simulink model "CopterSim3DEnvironment"  (R2017b)
settings: Solver=ode4  StartTime=0.0  StopTime=2000  FixedStep=0.001  RelTol=1e-3
PreLoadFcn:
  | filepath  = fileparts(get_param(bdroot, 'FileName'))
  | cd(filepath);
InitFcn:
  | if exist('Init_control.m','file')
  |      Init_control;
  | end
values from neighbouring files (symbols this model uses):
  Kd_RP_AgngleRate = 0.005    [Init_control.m]
  Kd_YAW_AngleRate = 0.05    [Init_control.m]
  Ki_RP_AgngleRate = 0.01    [Init_control.m]
  Ki_YAW_AngleRate = 0.8    [Init_control.m]
  Kp_RP_AgngleRate = 0.55    [Init_control.m]
  Kp_RP_ANGLE = 6.5    [Init_control.m]
  Kp_YAW_AngleRate = 3.2    [Init_control.m]
  MAX_CONTROL_ANGLE_RATE_Y = 90    [Init_control.m]
  MAX_CONTROL_ANGLE_RP = 45    [Init_control.m]
undefined symbols (not defined in the file or in its folder): earthRadius, KiPitchAttitude, KiRollAttitude, ModelInit_RPM, ModelParam_envAltitude, ModelParam_GlobalNoiseGainSwitch, ModelParam_GPSLatLong, ModelParam_motorCr, ModelParam_motorJm, ModelParam_motorMinThr, ModelParam_motorT, ModelParam_motorWb, ModelParam_rotorCm, ModelParam_rotorCt, ModelParam_uavCCm, ModelParam_uavCd, ModelParam_uavDearo, ModelParam_uavJ, ModelParam_uavMass, ModelParam_uavR, ModelParam_uavType, Receive, Send
libraries: simulink x6, aerolibfltsims x4, etargetslib x2, shared6dof x1, aerolibanimutils x1, dspnetwork x1
(part 1 of 2)
settings Model: SimulationMode=accelerator  Creator=dream  LastModifiedBy=dream
settings DebuggingCC: BusObjectLabelMismatch=error
settings CodeAppCC: StateflowObjectComments=on

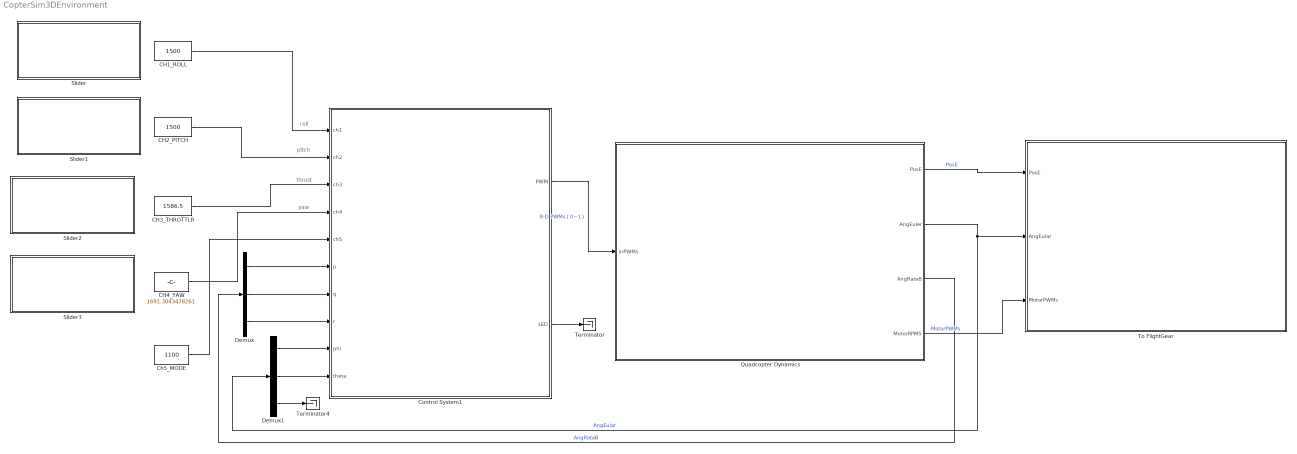
== system CopterSim3DEnvironment ==
  note: roll
  note: pitch
  note: thrust
  note: yaw
  "     CH3_THROTTLR " : Constant  Value=1586.5  OutDataTypeStr=uint16
  "     CH4_YAW     " : Constant  Value=1691.3043478261  OutDataTypeStr=uint16
  " CH2_PITCH " : Constant  Value=1500  OutDataTypeStr=uint16
  "CH1_ROLL   " : Constant  Value=1500  OutDataTypeStr=uint16
  "Ch5_MODE " : Constant  Value=1100  OutDataTypeStr=uint16
  Control System1 : Subsystem
      mask Display: image('icon\pixhawk.png');
  Demux : Demux  Outputs=3
  Demux1 : Demux  Outputs=3
  Quadcopter Dynamics : Subsystem
      mask Display: image('icon/F450.png');
  Slider : Subsystem  DialogController=hmiCreateDDGDialog  IsWebBlock=on  mask(MWDashboardBlock){webBlockId=da57f061-4e57-426f-be23-e227219c210b, webBlockType=slider, ShowInLibBrowser=on, ShowInitialText=on, HMISrcModelName=CopterSim3DEnvironment}
      mask prompts: webBlockId "WebBlock Id"; webBlockType "WebBlock Type"; HMISrcModelName "Source Model"
      mask help: SimulinkHMI:dialogs:SliderDialogDesc
      mask Help: helpview([docroot '/mapfiles/simulink.map'], 'hmi_slider')
      mask Display:
      | if strcmp(get_param(bdroot(gcb),'BlockDiagramType'), 'library')
      |     image([(matlabroot) '/toolbox/simulink/hmi/icons/Slider.png']);
      | end
  Slider1 : Subsystem  DialogController=hmiCreateDDGDialog  IsWebBlock=on  mask(MWDashboardBlock){webBlockId=f8138af1-f0d8-4bb2-b2ca-4a41ecd2e2bf, webBlockType=slider, ShowInLibBrowser=on, ShowInitialText=on, HMISrcModelName=CopterSim3DEnvironment}
      mask prompts: webBlockId "WebBlock Id"; webBlockType "WebBlock Type"; HMISrcModelName "Source Model"
      mask help: SimulinkHMI:dialogs:SliderDialogDesc
      mask Help: helpview([docroot '/mapfiles/simulink.map'], 'hmi_slider')
      mask Display:
      | if strcmp(get_param(bdroot(gcb),'BlockDiagramType'), 'library')
      |     image([(matlabroot) '/toolbox/simulink/hmi/icons/Slider.png']);
      | end
  Slider2 : Subsystem  DialogController=hmiCreateDDGDialog  IsWebBlock=on  mask(MWDashboardBlock){webBlockId=6ace0251-812b-4be1-a029-ff54be59cd06, webBlockType=slider, ShowInLibBrowser=on, ShowInitialText=on, HMISrcModelName=CopterSim3DEnvironment}
      mask prompts: webBlockId "WebBlock Id"; webBlockType "WebBlock Type"; HMISrcModelName "Source Model"
      mask help: SimulinkHMI:dialogs:SliderDialogDesc
      mask Help: helpview([docroot '/mapfiles/simulink.map'], 'hmi_slider')
      mask Display:
      | if strcmp(get_param(bdroot(gcb),'BlockDiagramType'), 'library')
      |     image([(matlabroot) '/toolbox/simulink/hmi/icons/Slider.png']);
      | end
  Slider3 : Subsystem  DialogController=hmiCreateDDGDialog  IsWebBlock=on  mask(MWDashboardBlock){webBlockId=7791c665-d291-46cf-a452-489177f2fb62, webBlockType=slider, ShowInLibBrowser=on, ShowInitialText=on, HMISrcModelName=CopterSim3DEnvironment}
      mask prompts: webBlockId "WebBlock Id"; webBlockType "WebBlock Type"; HMISrcModelName "Source Model"
      mask help: SimulinkHMI:dialogs:SliderDialogDesc
      mask Help: helpview([docroot '/mapfiles/simulink.map'], 'hmi_slider')
      mask Display:
      | if strcmp(get_param(bdroot(gcb),'BlockDiagramType'), 'library')
      |     image([(matlabroot) '/toolbox/simulink/hmi/icons/Slider.png']);
      | end
  Terminator : Terminator
  Terminator4 : Terminator
  To FlightGear : Subsystem
      mask Display: image('icon/FlightGear.png');
  wires:
  Quadcopter Dynamics/1(PosE) -> To FlightGear/1(PosE)  "PosE"
  Control System1/2(LED) -> Terminator/1
  Quadcopter Dynamics/2(AngEuler) -> To FlightGear/2(AngEular), Demux1/1  "AngEular"
  "CH1_ROLL   "/1 -> Control System1/1(ch1)
  "     CH4_YAW     "/1 -> Control System1/4(ch4)
  "     CH3_THROTTLR "/1 -> Control System1/3(ch3)
  Quadcopter Dynamics/3(AngRateB) -> Demux/1  "AngRateB"
  "Ch5_MODE "/1 -> Control System1/5(ch5)
  Demux/1 -> Control System1/6(p)
  Demux/2 -> Control System1/7(q)
  Demux/3 -> Control System1/8(r)
  Demux1/1 -> Control System1/9(phi)
  Demux1/2 -> Control System1/10(theta)
  Demux1/3 -> Terminator4/1
  " CH2_PITCH "/1 -> Control System1/2(ch2)
  Control System1/1(PWM) -> Quadcopter Dynamics/1(inPWMs)  "8-D PWMs（0~1）"
  Quadcopter Dynamics/4(MotorRPMS) -> To FlightGear/3(MotorPWMs)  "MotorPWMs"

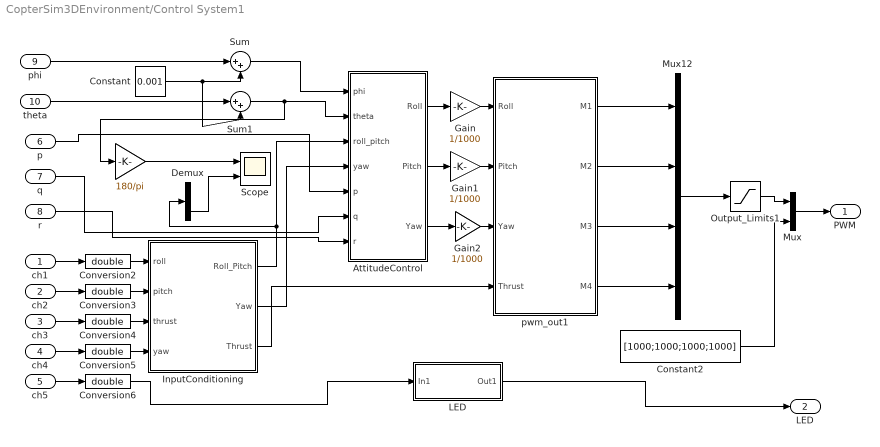
== system CopterSim3DEnvironment/Control System1 ==
  ch1 : Inport  OutDataTypeStr=uint16  PortDimensions=1
  ch2 : Inport  Port=2  OutDataTypeStr=uint16  PortDimensions=1
  ch3 : Inport  Port=3  OutDataTypeStr=uint16  PortDimensions=1
  ch4 : Inport  Port=4  OutDataTypeStr=uint16  PortDimensions=1
  ch5 : Inport  Port=5  OutDataTypeStr=uint16  PortDimensions=1  Interpolate=off
  p : Inport  Port=6  PortDimensions=1
  q : Inport  Port=7  PortDimensions=1
  r : Inport  Port=8  PortDimensions=1
  phi : Inport  Port=9  PortDimensions=1
  theta : Inport  Port=10  PortDimensions=1
  " " : Gain  Gain=180/pi
  AttitudeControl : Subsystem
  Constant : Constant  Value=0.001
  Constant2 : Constant  Value=[1000;1000;1000;1000]
  Conversion{2..6} (5 alike) : DataTypeConversion  OutDataTypeStr=double
  Demux : Demux  Outputs=2
  Gain : Gain  Gain=1/1000
  Gain1 : Gain  Gain=1/1000
  Gain2 : Gain  Gain=1/1000
  InputConditioning : Subsystem
  "LED " : Subsystem
  Mux : Mux  Inputs=2
  Mux12 : Mux
  Output_Limits1 : Saturate  UpperLimit=2000  LowerLimit=1000
  Scope : Scope  NumInputPorts=2
  Sum : Sum  Inputs=|++
  Sum1 : Sum  Inputs=|++
  pwm_out1 : MATLAB Function  TreatAsAtomicUnit=on  SystemSampleTime=0.004
  PWM : Outport  PortDimensions=8
  LED : Outport  Port=2  PortDimensions=1
  wires:
  InputConditioning/3(Thrust) -> pwm_out1/4(Thrust)
  Mux12/1 -> Output_Limits1/1
  Gain1/1 -> pwm_out1/2(Pitch)
  Gain/1 -> pwm_out1/1(Roll)
  ch3/1 -> Conversion4/1
  pwm_out1/1(M1) -> Mux12/1
  ch5/1 -> Conversion6/1
  pwm_out1/3(M3) -> Mux12/3
  pwm_out1/2(M2) -> Mux12/2
  r/1 -> AttitudeControl/7(r)
  AttitudeControl/1(Roll) -> Gain/1
  Gain2/1 -> pwm_out1/3(Yaw)
  InputConditioning/1(Roll_Pitch) -> Demux/1, AttitudeControl/3(roll_pitch)
  q/1 -> AttitudeControl/6(q)
  theta/1 -> Sum1/1
  InputConditioning/2(Yaw) -> AttitudeControl/4(yaw)
  p/1 -> AttitudeControl/5(p)
  ch4/1 -> Conversion5/1
  pwm_out1/4(M4) -> Mux12/4
  AttitudeControl/3(Yaw) -> Gain2/1
  AttitudeControl/2(Pitch) -> Gain1/1
  ch1/1 -> Conversion2/1
  "LED "/1(Out1) -> LED/1
  ch2/1 -> Conversion3/1
  Conversion6/1 -> "LED "/1(In1)
  Conversion2/1 -> InputConditioning/1(roll)
  Conversion5/1 -> InputConditioning/4(yaw)
  Conversion4/1 -> InputConditioning/3(thrust)
  Conversion3/1 -> InputConditioning/2(pitch)
  " "/1 -> Scope/1
  Demux/2 -> Scope/2
  phi/1 -> Sum/1
  Sum/1 -> AttitudeControl/1(phi)
  Sum1/1 -> " "/1, AttitudeControl/2(theta)
  Constant/1 -> Sum1/2, Sum/2
  Constant2/1 -> Mux/2
  Output_Limits1/1 -> Mux/1
  Mux/1 -> PWM/1

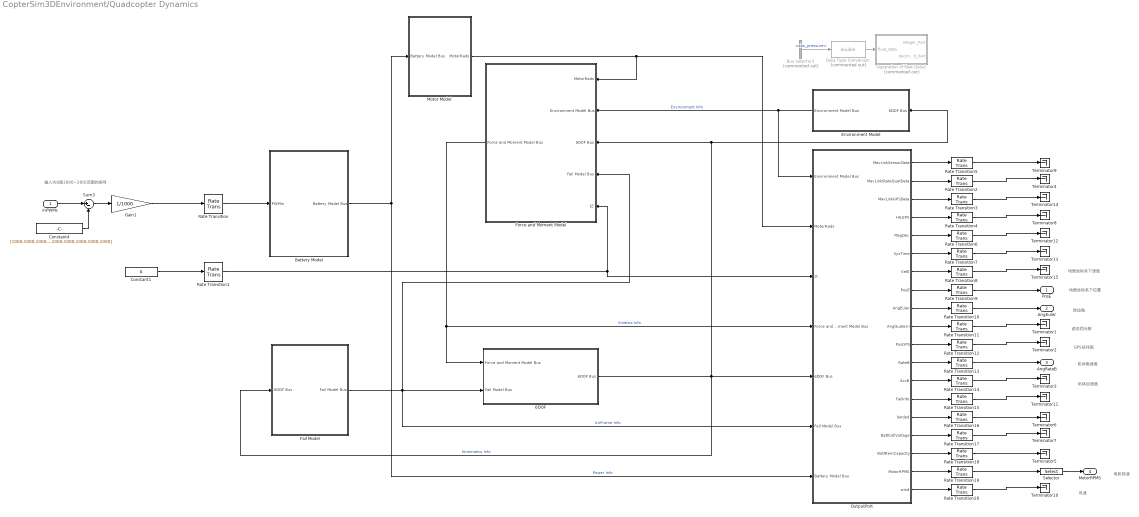
== system CopterSim3DEnvironment/Quadcopter Dynamics ==
  note: 电机转速
  note: 风速
  note: 机体加速度
  note: 机体角速度
  note: GPS经纬高
  note: 姿态四元数
  note: 欧拉角
  note: 地面坐标系下位置
  note: 地面坐标系下速度
  note: 输入为8路1000~2000范围的信号
  inPWMs : Inport  PortDimensions=8
  6DOF : Subsystem
  Battery Model : Subsystem
      mask help: Simulink:masks:GenSFuncDesc_MD
      mask Help: eval('feval(''rtwprivate'',''rtwhelpview'',''rtw_sfcn_block'')');
  Bus Selector3 : BusSelector  Commented=on  OutputSignals=abs_pressure
  Constant1 : Constant  Value=0
  Constant4 : Constant  Value=[1000;1000;1000;1000;1000;1000;1000;1000]
  Data Type Conversion : DataTypeConversion  Commented=on  OutDataTypeStr=double
  Environment Model : Subsystem  mask{sfcnParam1=ModelParam_GPSLatLong, sfcnParam2=ModelParam_GlobalNoiseGainSwitch, sfcnParam3=ModelParam_envAltitude}
      mask prompts: sfcnParam1 "ModelParam_GPSLatLong:"; sfcnParam2 "ModelParam_GlobalNoiseGainSwitch:"; sfcnParam3 "ModelParam_envAltitude:"
      mask help: Simulink:masks:GenSFuncDesc_MD
      mask Help: eval('feval(''rtwprivate'',''rtwhelpview'',''rtw_sfcn_block'')');
  Fail Model : Subsystem  mask{sfcnParam1=ModelParam_uavJ, sfcnParam2=ModelParam_uavMass, sfcnParam3=ModelParam_uavR}
      mask prompts: sfcnParam1 "ModelParam_uavJ:"; sfcnParam2 "ModelParam_uavMass:"; sfcnParam3 "ModelParam_uavR:"
      mask help: Simulink:masks:GenSFuncDesc_MD
      mask Help: eval('feval(''rtwprivate'',''rtwhelpview'',''rtw_sfcn_block'')');
  Force and Moment Model : Subsystem  mask{sfcnParam1=ModelParam_motorJm, sfcnParam2=ModelParam_rotorCm, sfcnParam3=ModelParam_rotorCt, sfcnParam4=ModelParam_uavCCm, sfcnParam5=ModelParam_uavCd, sfcnParam6=ModelParam_uavDearo, sfcnParam7=ModelParam_uavR, sfcnParam8=ModelParam_uavType}
      mask prompts: sfcnParam1 "ModelParam_motorJm:"; sfcnParam2 "ModelParam_rotorCm:"; sfcnParam3 "ModelParam_rotorCt:"; sfcnParam4 "ModelParam_uavCCm:"; sfcnParam5 "ModelParam_uavCd:"; sfcnParam6 "ModelParam_uavDearo:"; sfcnParam7 "ModelParam_uavR:"; sfcnParam8 "ModelParam_uavType:"
      mask help: Simulink:masks:GenSFuncDesc_MD
      mask Help: eval('feval(''rtwprivate'',''rtwhelpview'',''rtw_sfcn_block'')');
  Gain1 : Gain  Gain=1/1000
  Motor Model : Subsystem  mask{sfcnParam1=ModelInit_RPM, sfcnParam2=ModelParam_motorCr, sfcnParam3=ModelParam_motorMinThr, sfcnParam4=ModelParam_motorT, sfcnParam5=ModelParam_motorWb}
      mask prompts: sfcnParam1 "ModelInit_RPM:"; sfcnParam2 "ModelParam_motorCr:"; sfcnParam3 "ModelParam_motorMinThr:"; sfcnParam4 "ModelParam_motorT:"; sfcnParam5 "ModelParam_motorWb:"
      mask help: Simulink:masks:GenSFuncDesc_MD
      mask Help: eval('feval(''rtwprivate'',''rtwhelpview'',''rtw_sfcn_block'')');
  OutputPort : Subsystem  mask{sfcnParam1=ModelParam_GPSLatLong, sfcnParam2=ModelParam_GlobalNoiseGainSwitch, sfcnParam3=ModelParam_envAltitude}
      mask prompts: sfcnParam1 "ModelParam_GPSLatLong:"; sfcnParam2 "ModelParam_GlobalNoiseGainSwitch:"; sfcnParam3 "ModelParam_envAltitude:"
      mask help: Simulink:masks:GenSFuncDesc_MD
      mask Help: eval('feval(''rtwprivate'',''rtwhelpview'',''rtw_sfcn_block'')');
  Rate Transition{,1..20} (21 alike) : RateTransition  OutPortSampleTime=ModelParam_BusSampleRate
  Selector : Selector  InputPortWidth=8  IndexOptions=Index vector (dialog)  Indices=[1 2 3 4]  OutputSizes=1
  Separation of float Data1 : Subsystem  Commented=on  mask{IntUint=1}
      mask prompts: IntUint "整数单位"
      mask help: 分离浮点数的整数和小数部分，这样在Labview MIT模块中可以稳定输出精度
  Sum3 : Sum  Inputs=|+-
  Terminator{1..15} (15 alike) : Terminator
  PosE : Outport
  AngEuler : Outport  Port=2
  AngRateB : Outport  Port=3
  MotorRPMS : Outport  Port=4
  wires:
  Selector/1 -> MotorRPMS/1
  Constant4/1 -> Sum3/2
  inPWMs/1 -> Sum3/1
  Constant1/1 -> Rate Transition1/1
  Sum3/1 -> Gain1/1
  Rate Transition5/1 -> Terminator9/1
  Rate Transition2/1 -> Terminator4/1
  Rate Transition3/1 -> Terminator14/1
  Rate Transition4/1 -> Terminator8/1
  Rate Transition6/1 -> Terminator12/1
  Rate Transition7/1 -> Terminator13/1
  Rate Transition8/1 -> Terminator15/1
  Rate Transition9/1 -> PosE/1
  Rate Transition10/1 -> AngEuler/1
  Rate Transition11/1 -> Terminator1/1
  Rate Transition12/1 -> Terminator2/1
  Rate Transition13/1 -> AngRateB/1
  Rate Transition14/1 -> Terminator3/1
  Rate Transition15/1 -> Terminator11/1
  Rate Transition16/1 -> Terminator6/1
  Rate Transition17/1 -> Terminator7/1
  Rate Transition18/1 -> Terminator5/1
  Rate Transition19/1 -> Selector/1
  Rate Transition20/1 -> Terminator10/1
  Gain1/1 -> Rate Transition/1
  OutputPort/2(MavLinkStateQuatData) -> Rate Transition2/1
  Motor Model/1(MotorRads) -> OutputPort/2(MotorRads), Force and Moment Model/1(MotorRads)
  OutputPort/15(landed) -> Rate Transition16/1
  OutputPort/3(MavLinkGPSData) -> Rate Transition3/1
  Bus Selector3/1 -> Data Type Conversion/1  "<abs_pressure>"
  Data Type Conversion/1 -> Separation of float Data1/1(float_Data)
  OutputPort/1(MavLinkSensorData) -> Rate Transition5/1
  OutputPort/14(FailInfo) -> Rate Transition15/1
  OutputPort/13(AccB) -> Rate Transition14/1
  OutputPort/12(RateB) -> Rate Transition13/1
  OutputPort/11(PosGPS) -> Rate Transition12/1
  OutputPort/10(AngQuatern) -> Rate Transition11/1
  OutputPort/9(AngEuler) -> Rate Transition10/1
  OutputPort/8(PosE) -> Rate Transition9/1
  OutputPort/7(VelE) -> Rate Transition8/1
  OutputPort/6(SysTime) -> Rate Transition7/1
  OutputPort/5(MagDec) -> Rate Transition6/1
  OutputPort/4(HILGPS) -> Rate Transition4/1
  Battery Model/1(Battery Model Bus) -> OutputPort/7(Battery Model Bus), Motor Model/1(Battery Model Bus)  "Power Info"
  Fail Model/1(Fail Model Bus) -> OutputPort/6(Fail Model Bus), Force and Moment Model/4(Fail Model Bus), 6DOF/2(Fail Model Bus)  "AirFrame Info"
  Force and Moment Model/1(Force and Moment Model Bus) -> OutputPort/4(Force and Moment Model Bus), 6DOF/1(Force and Moment Model Bus)  "Kinetics Info"
  6DOF/1(6DOF Bus) -> OutputPort/5(6DOF Bus), Fail Model/1(6DOF Bus), Environment Model/1(6DOF Bus), Force and Moment Model/3(6DOF Bus)  "Kinematics Info"
  Environment Model/1(Environment Model Bus) -> OutputPort/1(Environment Model Bus), Force and Moment Model/2(Environment Model Bus)  "Environment Info"
  OutputPort/16(BattCellVoltage) -> Rate Transition17/1
  OutputPort/17(BattRemCapacity) -> Rate Transition18/1
  OutputPort/19(wind) -> Rate Transition20/1
  OutputPort/18(MotorRPMS) -> Rate Transition19/1
  Rate Transition/1 -> Battery Model/1(PWMin)
  Rate Transition1/1 -> OutputPort/3(zt), Force and Moment Model/5("tZ ")

== system CopterSim3DEnvironment/Slider ==

== system CopterSim3DEnvironment/Slider1 ==

== system CopterSim3DEnvironment/Slider2 ==

== system CopterSim3DEnvironment/Slider3 ==

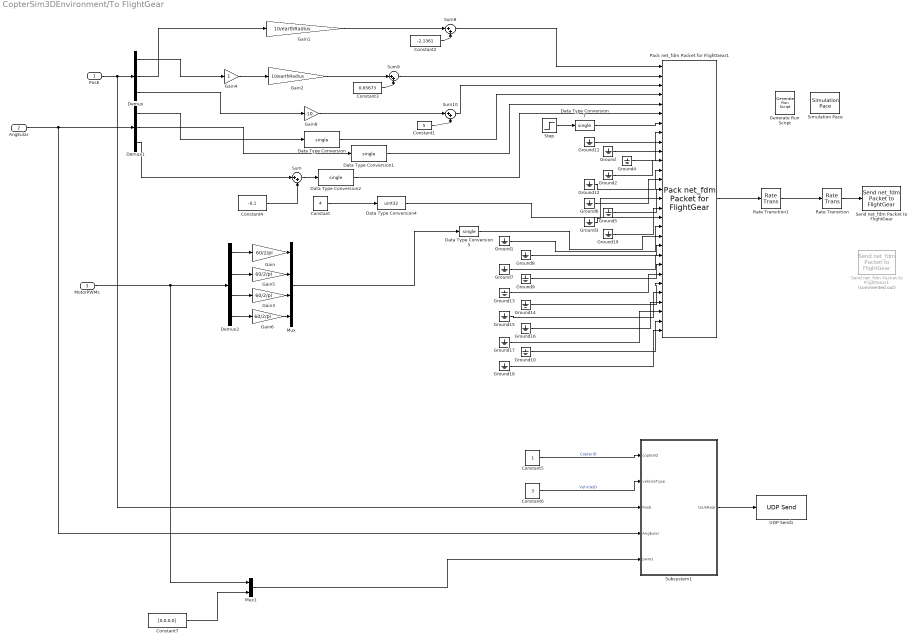
== system CopterSim3DEnvironment/To FlightGear ==
  PosE : Inport
  AngEular : Inport  Port=2
  MotorPWMs : Inport  Port=3
  Constant : Constant  Value=4
  Constant1 : Constant  Value=5  VectorParams1D=off
  Constant2 : Constant  Value=-2.1361  VectorParams1D=off
  Constant3 : Constant  Value=0.65673  VectorParams1D=off
  Constant4 : Constant  Value=-0.1  VectorParams1D=off
  Constant5 : Constant
  Constant6 : Constant  Value=3
  Constant7 : Constant  Value=[0,0,0,0]
  Data Type Conversion : DataTypeConversion  OutDataTypeStr=single  SaturateOnIntegerOverflow=on
  Data Type Conversion1 : DataTypeConversion  OutDataTypeStr=single  SaturateOnIntegerOverflow=on
  Data Type Conversion2 : DataTypeConversion  OutDataTypeStr=single  SaturateOnIntegerOverflow=on
  Data Type Conversion4 : DataTypeConversion  OutDataTypeStr=uint32
  Data Type Conversion5 : DataTypeConversion  OutDataTypeStr=single
  Data Type Conversion7 : DataTypeConversion  OutDataTypeStr=single
  Demux : Demux  Outputs=3
  Demux1 : Demux  Outputs=3
  Demux2 : Demux
  Gain{,3,5..6} (4 alike) : Gain  Gain=60/2/pi
  Gain1 : Gain  Gain=10/earthRadius
  Gain2 : Gain  Gain=10/earthRadius
  Gain4 : Gain
  Gain8 : Gain  Gain=-10
  Generate Run Script : aerolibfltsims/Generate Run Script  OutputFileName=runfg.bat  FlightGearBaseDirectory=C:\Program Files\FlightGear 2016.1.2  GeometryModelName=Rotor4  DestinationPort=5502  OriginAddress=127.0.0.1  OriginPort=5505  LocalAddress=127.0.0.1  AirportId=KSF0  RunwayId=10L  InitialAltitude=0  InitialHeading=0  OffsetDistance=0  OffsetAzimuth=0  GenerateFile=off  Architecture=Default  dataFlow=Send-Receive
  Ground{,1..19} (20 alike) : Ground
  Mux : Mux
  Mux1 : Mux  Inputs=2
  Pack net_fdm Packet for FlightGear1 : aerolibfltsims/Pack net_fdm Packet for FlightGear  FlightGearVersion=v2016.1  ShowPositionAttitudeInputs=on  ShowVelocityAccelerationInputs=off  ShowControlSurfacePositionInputs=on  ShowEngineFuelInputs=on  ShowLandingGearInputs=off  ShowEnvironmentInputs=off  SampleTime=0.01
      settings: SourceProductName=Aerospace Blockset  SourceProductBaseCode=AE
  Rate Transition : RateTransition
  Rate Transition1 : RateTransition
  Send net_fdm Packet to FlightGear : aerolibfltsims/Send net_fdm Packet to FlightGear  DestinationIpAddress=127.0.0.1  DestinationPort=5502  LocalIpPort=-1  varLen=off  SampleTime=0.005
      settings: SourceProductName=Aerospace Blockset  SourceProductBaseCode=AE
  Send net_fdm Packet to FlightGear1 : aerolibfltsims/Send net_fdm Packet to FlightGear  Commented=on  DestinationIpAddress=192.168.199.46  DestinationPort=5502  LocalIpPort=-1  varLen=off  SampleTime=0.01
      settings: SourceProductName=Aerospace Blockset  SourceProductBaseCode=AE
  Simulation Pace : aerolibanimutils/Simulation Pace  SimulationPace=1  SleepMode=MATLAB Thread  OutputPaceError=off  SampleTime=-1
      settings: AttributesFormatString=%<SimulationPace> sec/sec
  Step : Step  Time=5  SampleTime=0
  Subsystem1 : Subsystem
  Sum{,8..10} (4 alike) : Sum  Inputs=|++
  UDP Send1 : dspnetwork/UDP Send  remoteURL='127.0.0.1'  remotePort=20010  localURL='0.0.0.0'  localPortSource=Automatically determine  localPort=-1  sampletime=-1  blockPlatform=[]  separateLengthPort=0
      settings: SourceProductName=DSP System Toolbox  SourceProductBaseCode=DS
  wires:
  Rate Transition/1 -> Send net_fdm Packet to FlightGear/1
  Demux/1 -> Gain4/1
  Demux/2 -> Gain1/1
  Demux/3 -> Gain8/1
  Constant4/1 -> Sum/2
  Sum/1 -> Data Type Conversion2/1
  Gain1/1 -> Sum8/1
  Constant2/1 -> Sum8/2
  Gain2/1 -> Sum9/1
  Constant3/1 -> Sum9/2
  Constant1/1 -> Sum10/2
  Gain8/1 -> Sum10/1
  Pack net_fdm Packet for FlightGear1/1 -> Rate Transition1/1
  Demux1/2 -> Data Type Conversion1/1
  Demux1/3 -> Sum/1
  Data Type Conversion7/1 -> Pack net_fdm Packet for FlightGear1/7
  Ground8/1 -> Pack net_fdm Packet for FlightGear1/20
  Ground/1 -> Pack net_fdm Packet for FlightGear1/9
  Ground7/1 -> Pack net_fdm Packet for FlightGear1/21
  Ground9/1 -> Pack net_fdm Packet for FlightGear1/22
  Ground13/1 -> Pack net_fdm Packet for FlightGear1/23
  Ground14/1 -> Pack net_fdm Packet for FlightGear1/24
  Ground15/1 -> Pack net_fdm Packet for FlightGear1/25
  Ground16/1 -> Pack net_fdm Packet for FlightGear1/26
  Ground17/1 -> Pack net_fdm Packet for FlightGear1/27
  Ground10/1 -> Pack net_fdm Packet for FlightGear1/28
  Ground18/1 -> Pack net_fdm Packet for FlightGear1/29
  Step/1 -> Data Type Conversion7/1
  Data Type Conversion4/1 -> Pack net_fdm Packet for FlightGear1/17
  Ground1/1 -> Pack net_fdm Packet for FlightGear1/18
  Ground3/1 -> Pack net_fdm Packet for FlightGear1/15
  Ground5/1 -> Pack net_fdm Packet for FlightGear1/14
  Ground6/1 -> Pack net_fdm Packet for FlightGear1/13
  Ground4/1 -> Pack net_fdm Packet for FlightGear1/10
  Ground11/1 -> Pack net_fdm Packet for FlightGear1/8
  Data Type Conversion2/1 -> Pack net_fdm Packet for FlightGear1/6
  Data Type Conversion1/1 -> Pack net_fdm Packet for FlightGear1/5
  Data Type Conversion/1 -> Pack net_fdm Packet for FlightGear1/4
  Sum8/1 -> Pack net_fdm Packet for FlightGear1/1
  Sum9/1 -> Pack net_fdm Packet for FlightGear1/2
  Sum10/1 -> Pack net_fdm Packet for FlightGear1/3
  Constant/1 -> Data Type Conversion4/1
  Data Type Conversion5/1 -> Pack net_fdm Packet for FlightGear1/19
  Ground2/1 -> Pack net_fdm Packet for FlightGear1/11
  Ground12/1 -> Pack net_fdm Packet for FlightGear1/12
  Ground19/1 -> Pack net_fdm Packet for FlightGear1/16
  Gain4/1 -> Gain2/1
  MotorPWMs/1 -> Mux1/1, Demux2/1
  Mux/1 -> Data Type Conversion5/1
  Demux2/1 -> Gain/1
  Demux2/3 -> Gain3/1
  Gain/1 -> Mux/1
  Gain3/1 -> Mux/3
  Demux2/2 -> Gain5/1
  Gain5/1 -> Mux/2
  Demux2/4 -> Gain6/1
  Gain6/1 -> Mux/4
  Demux1/1 -> Data Type Conversion/1
  Rate Transition1/1 -> Rate Transition/1
  Constant6/1 -> Subsystem1/2(vehicleType)  "VehicleID"
  PosE/1 -> Subsystem1/3(PosE), Demux/1
  Constant5/1 -> Subsystem1/1(copterID)  "CopterID"
  Subsystem1/1(toUnReal) -> UDP Send1/1
  AngEular/1 -> Demux1/1, Subsystem1/4(AngEuler)
  Constant7/1 -> Mux1/2
  Mux1/1 -> Subsystem1/5(pwms)

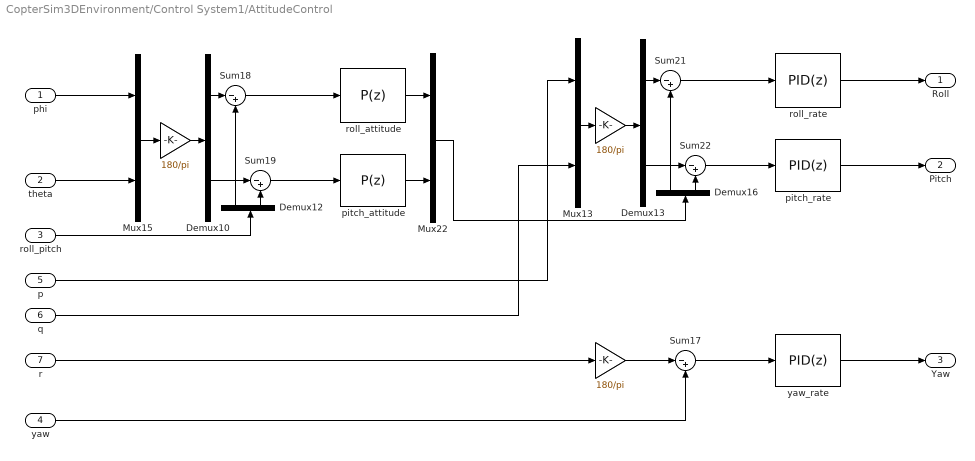
== system CopterSim3DEnvironment/Control System1/AttitudeControl ==
  phi : Inport
  theta : Inport  Port=2
  roll_pitch : Inport  Port=3
  yaw : Inport  Port=4
  p : Inport  Port=5
  q : Inport  Port=6
  r : Inport  Port=7
  " " : Gain  Gain=180/pi
  "  " : Gain  Gain=180/pi
  "          " : Gain  Gain=180/pi
  Demux{10,12..13,16} (4 alike) : Demux  Outputs=2
  Mux13 : Mux  Inputs=2
  Mux15 : Mux  Inputs=2
  Mux22 : Mux  Inputs=2
  Sum{17..19,21..22} (5 alike) : Sum  Inputs=|-+
  pitch_attitude : simulink/Continuous/PID Controller  Controller=P  TimeDomain=Discrete-time  SampleTime=-1  IntegratorMethod=Forward Euler  FilterMethod=Forward Euler  Form=Parallel  UseFilter=on  ControllerParametersSource=internal  P=Kp_RP_ANGLE  I=KiPitchAttitude  D=0.01  N=100  InitialConditionSource=internal  InitialConditionForIntegrator=0  InitialConditionForFilter=0  ExternalReset=none  LimitOutput=on  UpperSaturationLimit=180  LowerSaturationLimit=-180  LinearizeAsGain=on  AntiWindupMode=back-calculation  Kb=1  TrackingMode=off  Kt=1  PParamMin=[]  PParamMax=[]  IParamMin=[]  IParamMax=[]  DParamMin=[]  DParamMax=[]  NParamMin=[]  NParamMax=[]  KbParamMin=[]  KbParamMax=[]  KtParamMin=[]  KtParamMax=[]  POutMin=[]  POutMax=[]  IOutMin=[]  IOutMax=[]  DOutMin=[]  DOutMax=[]  NOutMin=[]  NOutMax=[]  KbOutMin=[]  KbOutMax=[]  KtOutMin=[]  KtOutMax=[]  IntegratorOutMin=[]  IntegratorOutMax=[]  FilterOutMin=[]  FilterOutMax=[]  SumOutMin=[]  SumOutMax=[]  SumI1OutMin=[]  SumI1OutMax=[]  SumI2OutMin=[]  SumI2OutMax=[]  SumI3OutMin=[]  SumI3OutMax=[]  SumDOutMin=[]  SumDOutMax=[]  SaturationOutMin=[]  SaturationOutMax=[]  IntegratorContinuousStateAttributes=''  IntegratorStateMustResolveToSignalObject=off  IntegratorRTWStateStorageClass=Auto  FilterContinuousStateAttributes=''  FilterStateMustResolveToSignalObject=off  FilterRTWStateStorageClass=Auto  DifferentiatorICPrevScaledInput=0  DifferentiatorOutMin=[]  DifferentiatorOutMax=[]  InitialConditionSetting=State (most efficient)  FilterDiffOutCoefMin=[]  FilterDiffOutCoefMax=[]  SumDenOutMin=[]  SumDenOutMax=[]  SumNumOutMin=[]  SumNumOutMax=[]  ReciprocalOutMin=[]  ReciprocalOutMax=[]  DivideOutMin=[]  DivideOutMax=[]  TunerSelectOption=Transfer Function Based (PID Tuner App)
  pitch_rate : simulink/Continuous/PID Controller  Controller=PID  TimeDomain=Discrete-time  SampleTime=-1  IntegratorMethod=Forward Euler  FilterMethod=Forward Euler  Form=Parallel  UseFilter=off  ControllerParametersSource=internal  P=Kp_RP_AgngleRate  I=Ki_RP_AgngleRate  D=Kd_RP_AgngleRate  N=100  InitialConditionSource=internal  InitialConditionForIntegrator=0  InitialConditionForFilter=0  ExternalReset=none  LimitOutput=on  UpperSaturationLimit=500  LowerSaturationLimit=-500  LinearizeAsGain=on  AntiWindupMode=back-calculation  Kb=1  TrackingMode=off  Kt=1  PParamMin=[]  PParamMax=[]  IParamMin=[]  IParamMax=[]  DParamMin=[]  DParamMax=[]  NParamMin=[]  NParamMax=[]  KbParamMin=[]  KbParamMax=[]  KtParamMin=[]  KtParamMax=[]  POutMin=[]  POutMax=[]  IOutMin=[]  IOutMax=[]  DOutMin=[]  DOutMax=[]  NOutMin=[]  NOutMax=[]  KbOutMin=[]  KbOutMax=[]  KtOutMin=[]  KtOutMax=[]  IntegratorOutMin=[]  IntegratorOutMax=[]  FilterOutMin=[]  FilterOutMax=[]  SumOutMin=[]  SumOutMax=[]  SumI1OutMin=[]  SumI1OutMax=[]  SumI2OutMin=[]  SumI2OutMax=[]  SumI3OutMin=[]  SumI3OutMax=[]  SumDOutMin=[]  SumDOutMax=[]  SaturationOutMin=[]  SaturationOutMax=[]  IntegratorContinuousStateAttributes=''  IntegratorStateMustResolveToSignalObject=off  IntegratorRTWStateStorageClass=Auto  FilterContinuousStateAttributes=''  FilterStateMustResolveToSignalObject=off  FilterRTWStateStorageClass=Auto  DifferentiatorICPrevScaledInput=0  DifferentiatorOutMin=[]  DifferentiatorOutMax=[]  InitialConditionSetting=State (most efficient)  FilterDiffOutCoefMin=[]  FilterDiffOutCoefMax=[]  SumDenOutMin=[]  SumDenOutMax=[]  SumNumOutMin=[]  SumNumOutMax=[]  ReciprocalOutMin=[]  ReciprocalOutMax=[]  DivideOutMin=[]  DivideOutMax=[]  TunerSelectOption=Transfer Function Based (PID Tuner App)
  roll_attitude : simulink/Continuous/PID Controller  Controller=P  TimeDomain=Discrete-time  SampleTime=-1  IntegratorMethod=Forward Euler  FilterMethod=Forward Euler  Form=Parallel  UseFilter=on  ControllerParametersSource=internal  P=Kp_RP_ANGLE  I=KiRollAttitude  D=0.01  N=100  InitialConditionSource=internal  InitialConditionForIntegrator=0  InitialConditionForFilter=0  ExternalReset=none  LimitOutput=on  UpperSaturationLimit=180  LowerSaturationLimit=-180  LinearizeAsGain=on  AntiWindupMode=back-calculation  Kb=1  TrackingMode=off  Kt=1  PParamMin=[]  PParamMax=[]  IParamMin=[]  IParamMax=[]  DParamMin=[]  DParamMax=[]  NParamMin=[]  NParamMax=[]  KbParamMin=[]  KbParamMax=[]  KtParamMin=[]  KtParamMax=[]  POutMin=[]  POutMax=[]  IOutMin=[]  IOutMax=[]  DOutMin=[]  DOutMax=[]  NOutMin=[]  NOutMax=[]  KbOutMin=[]  KbOutMax=[]  KtOutMin=[]  KtOutMax=[]  IntegratorOutMin=[]  IntegratorOutMax=[]  FilterOutMin=[]  FilterOutMax=[]  SumOutMin=[]  SumOutMax=[]  SumI1OutMin=[]  SumI1OutMax=[]  SumI2OutMin=[]  SumI2OutMax=[]  SumI3OutMin=[]  SumI3OutMax=[]  SumDOutMin=[]  SumDOutMax=[]  SaturationOutMin=[]  SaturationOutMax=[]  IntegratorContinuousStateAttributes=''  IntegratorStateMustResolveToSignalObject=off  IntegratorRTWStateStorageClass=Auto  FilterContinuousStateAttributes=''  FilterStateMustResolveToSignalObject=off  FilterRTWStateStorageClass=Auto  DifferentiatorICPrevScaledInput=0  DifferentiatorOutMin=[]  DifferentiatorOutMax=[]  InitialConditionSetting=State (most efficient)  FilterDiffOutCoefMin=[]  FilterDiffOutCoefMax=[]  SumDenOutMin=[]  SumDenOutMax=[]  SumNumOutMin=[]  SumNumOutMax=[]  ReciprocalOutMin=[]  ReciprocalOutMax=[]  DivideOutMin=[]  DivideOutMax=[]  TunerSelectOption=Transfer Function Based (PID Tuner App)
  roll_rate : simulink/Continuous/PID Controller  Controller=PID  TimeDomain=Discrete-time  SampleTime=-1  IntegratorMethod=Forward Euler  FilterMethod=Forward Euler  Form=Parallel  UseFilter=off  ControllerParametersSource=internal  P=Kp_RP_AgngleRate  I=Ki_RP_AgngleRate  D=Kd_RP_AgngleRate  N=100  InitialConditionSource=internal  InitialConditionForIntegrator=0  InitialConditionForFilter=0  ExternalReset=none  LimitOutput=on  UpperSaturationLimit=500  LowerSaturationLimit=-500  LinearizeAsGain=on  AntiWindupMode=back-calculation  Kb=1  TrackingMode=off  Kt=1  PParamMin=[]  PParamMax=[]  IParamMin=[]  IParamMax=[]  DParamMin=[]  DParamMax=[]  NParamMin=[]  NParamMax=[]  KbParamMin=[]  KbParamMax=[]  KtParamMin=[]  KtParamMax=[]  POutMin=[]  POutMax=[]  IOutMin=[]  IOutMax=[]  DOutMin=[]  DOutMax=[]  NOutMin=[]  NOutMax=[]  KbOutMin=[]  KbOutMax=[]  KtOutMin=[]  KtOutMax=[]  IntegratorOutMin=[]  IntegratorOutMax=[]  FilterOutMin=[]  FilterOutMax=[]  SumOutMin=[]  SumOutMax=[]  SumI1OutMin=[]  SumI1OutMax=[]  SumI2OutMin=[]  SumI2OutMax=[]  SumI3OutMin=[]  SumI3OutMax=[]  SumDOutMin=[]  SumDOutMax=[]  SaturationOutMin=[]  SaturationOutMax=[]  IntegratorContinuousStateAttributes=''  IntegratorStateMustResolveToSignalObject=off  IntegratorRTWStateStorageClass=Auto  FilterContinuousStateAttributes=''  FilterStateMustResolveToSignalObject=off  FilterRTWStateStorageClass=Auto  DifferentiatorICPrevScaledInput=0  DifferentiatorOutMin=[]  DifferentiatorOutMax=[]  InitialConditionSetting=State (most efficient)  FilterDiffOutCoefMin=[]  FilterDiffOutCoefMax=[]  SumDenOutMin=[]  SumDenOutMax=[]  SumNumOutMin=[]  SumNumOutMax=[]  ReciprocalOutMin=[]  ReciprocalOutMax=[]  DivideOutMin=[]  DivideOutMax=[]  TunerSelectOption=Transfer Function Based (PID Tuner App)
  yaw_rate : simulink/Continuous/PID Controller  Controller=PID  TimeDomain=Discrete-time  SampleTime=-1  IntegratorMethod=Forward Euler  FilterMethod=Forward Euler  Form=Parallel  UseFilter=off  ControllerParametersSource=internal  P=Kp_YAW_AngleRate  I=Ki_YAW_AngleRate  D=Kd_YAW_AngleRate  N=100  InitialConditionSource=internal  InitialConditionForIntegrator=0  InitialConditionForFilter=0  ExternalReset=none  LimitOutput=on  UpperSaturationLimit=500  LowerSaturationLimit=-500  LinearizeAsGain=on  AntiWindupMode=back-calculation  Kb=1  TrackingMode=off  Kt=1  PParamMin=[]  PParamMax=[]  IParamMin=[]  IParamMax=[]  DParamMin=[]  DParamMax=[]  NParamMin=[]  NParamMax=[]  KbParamMin=[]  KbParamMax=[]  KtParamMin=[]  KtParamMax=[]  POutMin=[]  POutMax=[]  IOutMin=[]  IOutMax=[]  DOutMin=[]  DOutMax=[]  NOutMin=[]  NOutMax=[]  KbOutMin=[]  KbOutMax=[]  KtOutMin=[]  KtOutMax=[]  IntegratorOutMin=[]  IntegratorOutMax=[]  FilterOutMin=[]  FilterOutMax=[]  SumOutMin=[]  SumOutMax=[]  SumI1OutMin=[]  SumI1OutMax=[]  SumI2OutMin=[]  SumI2OutMax=[]  SumI3OutMin=[]  SumI3OutMax=[]  SumDOutMin=[]  SumDOutMax=[]  SaturationOutMin=[]  SaturationOutMax=[]  IntegratorContinuousStateAttributes=''  IntegratorStateMustResolveToSignalObject=off  IntegratorRTWStateStorageClass=Auto  FilterContinuousStateAttributes=''  FilterStateMustResolveToSignalObject=off  FilterRTWStateStorageClass=Auto  DifferentiatorICPrevScaledInput=0  DifferentiatorOutMin=[]  DifferentiatorOutMax=[]  InitialConditionSetting=State (most efficient)  FilterDiffOutCoefMin=[]  FilterDiffOutCoefMax=[]  SumDenOutMin=[]  SumDenOutMax=[]  SumNumOutMin=[]  SumNumOutMax=[]  ReciprocalOutMin=[]  ReciprocalOutMax=[]  DivideOutMin=[]  DivideOutMax=[]  TunerSelectOption=Transfer Function Based (PID Tuner App)
  Roll : Outport
  Pitch : Outport  Port=2
  Yaw : Outport  Port=3
  wires:
  r/1 -> "          "/1
  q/1 -> Mux13/2
  Mux22/1 -> Demux16/1
  yaw_rate/1 -> Yaw/1
  phi/1 -> Mux15/1
  Mux15/1 -> " "/1
  theta/1 -> Mux15/2
  "          "/1 -> Sum17/1
  roll_rate/1 -> Roll/1
  Sum19/1 -> pitch_attitude/1
  pitch_attitude/1 -> Mux22/2
  roll_attitude/1 -> Mux22/1
  Demux16/1 -> Sum21/2
  yaw/1 -> Sum17/2
  roll_pitch/1 -> Demux12/1
  Demux16/2 -> Sum22/2
  Demux12/1 -> Sum18/2
  Demux12/2 -> Sum19/2
  p/1 -> Mux13/1
  Demux10/1 -> Sum18/1
  Demux10/2 -> Sum19/1
  " "/1 -> Demux10/1
  Sum18/1 -> roll_attitude/1
  pitch_rate/1 -> Pitch/1
  Mux13/1 -> "  "/1
  Sum22/1 -> pitch_rate/1
  Sum17/1 -> yaw_rate/1
  Demux13/1 -> Sum21/1
  Demux13/2 -> Sum22/1
  "  "/1 -> Demux13/1
  Sum21/1 -> roll_rate/1

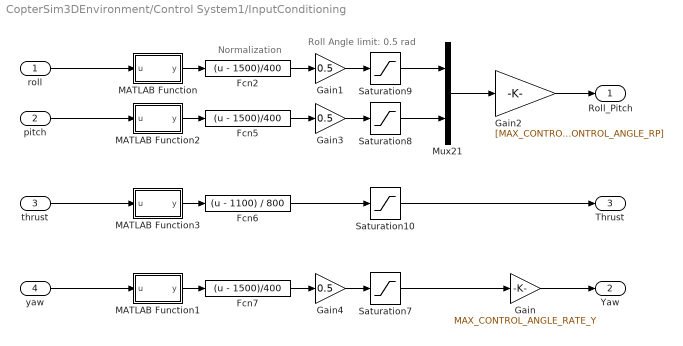
== system CopterSim3DEnvironment/Control System1/InputConditioning ==
  note: Roll Angle limit: 0.5 rad
  note: Normalization
  roll : Inport
  pitch : Inport  Port=2
  thrust : Inport  Port=3
  yaw : Inport  Port=4
  Fcn2 : Fcn  Expr=(u - 1500)/400
  Fcn5 : Fcn  Expr=(u - 1500)/400
  Fcn6 : Fcn  Expr=(u - 1100) / 800
  Fcn7 : Fcn  Expr=(u - 1500)/400
  Gain : Gain  Gain=MAX_CONTROL_ANGLE_RATE_Y
  Gain1 : Gain  Gain=0.5
  Gain2 : Gain  Gain=[MAX_CONTROL_ANGLE_RP MAX_CONTROL_ANGLE_RP]  OutDataTypeStr=Inherit: Inherit via back propagation
  Gain3 : Gain  Gain=0.5
  Gain4 : Gain  Gain=0.5
  MATLAB Function : MATLAB Function  TreatAsAtomicUnit=on
  MATLAB Function1 : MATLAB Function  TreatAsAtomicUnit=on
  MATLAB Function2 : MATLAB Function  TreatAsAtomicUnit=on
  MATLAB Function3 : MATLAB Function  TreatAsAtomicUnit=on
  Mux21 : Mux  Inputs=2
  Saturation10 : Saturate  UpperLimit=1  LowerLimit=0
  Saturation7 : Saturate  UpperLimit=1  LowerLimit=-1
  Saturation8 : Saturate  UpperLimit=1  LowerLimit=-1
  Saturation9 : Saturate  UpperLimit=1  LowerLimit=-1
  Roll_Pitch : Outport
  Yaw : Outport  Port=2
  Thrust : Outport  Port=3
  wires:
  Saturation10/1 -> Thrust/1
  Saturation7/1 -> Gain/1
  Gain2/1 -> Roll_Pitch/1
  Mux21/1 -> Gain2/1
  Saturation8/1 -> Mux21/2
  Fcn6/1 -> Saturation10/1
  Fcn2/1 -> Gain1/1
  Fcn5/1 -> Gain3/1
  Saturation9/1 -> Mux21/1
  Fcn7/1 -> Gain4/1
  pitch/1 -> MATLAB Function2/1(u)
  MATLAB Function1/1(y) -> Fcn7/1
  thrust/1 -> MATLAB Function3/1(u)
  roll/1 -> MATLAB Function/1(u)
  MATLAB Function2/1(y) -> Fcn5/1
  MATLAB Function/1(y) -> Fcn2/1
  yaw/1 -> MATLAB Function1/1(u)
  MATLAB Function3/1(y) -> Fcn6/1
  Gain/1 -> Yaw/1
  Gain1/1 -> Saturation9/1
  Gain3/1 -> Saturation8/1
  Gain4/1 -> Saturation7/1

== system CopterSim3DEnvironment/Control System1/LED  ==
  In1 : Inport
  Compare To Constant3 : simulink/Logic and Bit Operations/Compare To Constant  relop=>=  const=uint16(1500)  OutDataTypeStr=boolean
  Out1 : Outport
  wires:
  Compare To Constant3/1 -> Out1/1
  In1/1 -> Compare To Constant3/1

== system CopterSim3DEnvironment/Quadcopter Dynamics/6DOF ==
  Force and Moment Model Bus : Inport
  Fail Model Bus : Inport  Port=2
  Bus Creator : BusCreator  Inputs=7
  Bus Selector : BusSelector  OutputSignals=dM,m,J
  Bus Selector1 : BusSelector  OutputSignals=Fb,Mb
  Constant_dI/dt : Constant  Value=zeros(3,3)
  Custom Variable Mass 6DOF (Quaternion) : shared6dof/6DOF (Euler Angles)  units=Metric (MKS)  mtype=Custom Variable  rep=Quaternion  xme_0=ModelInit_PosE  Vm_0=ModelInit_VelB  eul_0=ModelInit_AngEuler  pm_0=ModelInit_RateB  mass_0=1.0  mass_e=0.5  mass_f=2.0  inertia=eye(3)  inertia_e=eye(3)  inertia_f=2*eye(3)  k_quat=1.0  vre_flag=off  abi_flag=off
      settings: SourceProductBaseCode=AE
  Sum : Sum  Inputs=++|
  Terminator : Terminator
  6DOF Bus : Outport
  wires:
  Bus Selector1/1 -> Custom Variable Mass 6DOF (Quaternion)/1  "<Fb>"
  Bus Selector/2 -> Custom Variable Mass 6DOF (Quaternion)/3  "<m>"
  Custom Variable Mass 6DOF (Quaternion)/8 -> Terminator/1
  Sum/1 -> Custom Variable Mass 6DOF (Quaternion)/2
  Constant_dI/dt/1 -> Custom Variable Mass 6DOF (Quaternion)/4
  Custom Variable Mass 6DOF (Quaternion)/5 -> Bus Creator/5  "Vb"
  Custom Variable Mass 6DOF (Quaternion)/6 -> Bus Creator/6  "wb"
  Custom Variable Mass 6DOF (Quaternion)/1 -> Bus Creator/1  "Ve"
  Custom Variable Mass 6DOF (Quaternion)/4 -> Bus Creator/4  "DCM"
  Custom Variable Mass 6DOF (Quaternion)/2 -> Bus Creator/2  "Xe"
  Custom Variable Mass 6DOF (Quaternion)/3 -> Bus Creator/3  "Eular(rad)"
  Custom Variable Mass 6DOF (Quaternion)/7 -> Bus Creator/7  "dwb/dt"
  Bus Selector/3 -> Custom Variable Mass 6DOF (Quaternion)/5  "<J>"
  Bus Selector/1 -> Sum/2  "<dM>"
  Bus Selector1/2 -> Sum/1  "<Mb>"
  Fail Model Bus/1 -> Bus Selector/1
  Force and Moment Model Bus/1 -> Bus Selector1/1
  Bus Creator/1 -> 6DOF Bus/1

== system CopterSim3DEnvironment/Quadcopter Dynamics/Battery Model ==
  PWMin : Inport
  Battery Model_sfcn : S-Function  FunctionName=Battery_sf  SFunctionModules=""  SFunctionDeploymentMode=off  EnableBusSupport=off  mask{rtw_sf_name=Battery_sf, showVar=off}
      mask prompts: rtw_sf_name "Simulink:masks:GenSFuncName_MP"; showVar "Simulink:masks:GenSFuncShowModuleList_MP"
      mask help: Simulink:masks:GenSFuncDesc_MD
      mask init:
      | displist = '';
      | if ~strcmp(get_param(gcb, 'FunctionName'), rtw_sf_name);
      |   set_param(gcb, 'FunctionName', rtw_sf_name);
      | end
      | % Check if we are generating code
      | rtw_mode = false;
      | if strcmpi(get_param(bdroot(gcb),'SimulationStatus'),'Initializing')
      | 	rtw_mode = strcmpi(get_param(bdroot(gcb),'BuildingRTWCode'),'on') && ...
      | 		~strcmpi(get_param(bdroot(gcb),'TargetStyle'),'SimulationTarget');
      | end
      | if showVar || rtw_mode
      | 	if exist('rtwsfunc') == 2 | exist('rtwsfunc') == 6
      | 		tmplist = rtwsfunc(rtw_sf_name,gcb);
      | 		tmplist = DAStudio.message('Simulink:masks:GenSFuncListOfModules_IC', tmplist);
      | 	elseif showVar
      | 		tmplist1 = DAStudio.message('Simulink:masks:GenSFuncListOfModules_IC', '');
      |         tmplist2 = DAStudio.message('Simulink:masks:GenSFuncNotLicensed_IC');
      |         tmplist = [tmplist1 tmplist2];
      |  	end
      | end
      | if showVar
      |   displist = tmplist;
      | end
      settings: CopyFcn=|
      | if ~strcmp(get_param(gcb,'Linkstatus'),'none') && ...
      | ~strcmp(get_param(gcb,'Linkstatus'),'implicit')
      |   set_param(gcb,'LinkStatus','none');
      | end
      mask Help: eval('feval(''rtwprivate'',''rtwhelpview'',''rtw_sfcn_block'')');
      mask Display:
      | port_label('input',1,'PWMin');
      | port_label('output',1,'PWMOut');
      | port_label('output',2,'cellVol');
      | port_label('output',3,'remCapa');
  __InputSSForSFun__ : Subsystem
  __OutputSSForSFun__ : Subsystem
  Battery Model Bus : Outport
  wires:
  PWMin/1 -> __InputSSForSFun__/1(PWMin)
  __InputSSForSFun__/1(__UniqueOutportName__1__) -> Battery Model_sfcn/1
  Battery Model_sfcn/1 -> __OutputSSForSFun__/1(__UniqueInportName__1__)
  Battery Model_sfcn/2 -> __OutputSSForSFun__/2(__UniqueInportName__2__)
  Battery Model_sfcn/3 -> __OutputSSForSFun__/3(__UniqueInportName__3__)
  __OutputSSForSFun__/1(Battery Model Bus) -> Battery Model Bus/1

== system CopterSim3DEnvironment/Quadcopter Dynamics/Environment Model ==
  6DOF Bus : Inport
  Environment Model_sfcn : S-Function  FunctionName=Environment_sf  Parameters=sfcnParam1, sfcnParam2, sfcnParam3  SFunctionModules=""  SFunctionDeploymentMode=off  EnableBusSupport=off  SFcnStateName=DWORK0  mask{rtw_sf_name=Environment_sf, showVar=off, sfcnParam1=sfcnParam1, sfcnParam2=sfcnParam2, sfcnParam3=sfcnParam3}
      mask prompts: rtw_sf_name "Simulink:masks:GenSFuncName_MP"; showVar "Simulink:masks:GenSFuncShowModuleList_MP"; sfcnParam1 "ModelParam_GPSLatLong:"; sfcnParam2 "ModelParam_GlobalNoiseGainSwitch:"; sfcnParam3 "ModelParam_envAltitude:"
      mask help: Simulink:masks:GenSFuncDesc_MD
      mask init: same as CopterSim3DEnvironment/Quadcopter Dynamics/Battery Model/Battery Model_sfcn
      settings: SFcnIsStateOwnerBlock=on
      settings: CopyFcn=|
      | if ~strcmp(get_param(gcb,'Linkstatus'),'none') && ...
      | ~strcmp(get_param(gcb,'Linkstatus'),'implicit')
      |   set_param(gcb,'LinkStatus','none');
      | end
      mask Help: eval('feval(''rtwprivate'',''rtwhelpview'',''rtw_sfcn_block'')');
      mask Display:
      | port_label('input',1,'Ve');
      | port_label('input',2,'Xe');
      | port_label('input',3,'Eular(rad)');
      | port_label('input',4,'DCM');
      | port_label('input',5,'Vb');
      | port_label('input',6,'wb');
      | port_label('input',7,'dwb/dt');
      | port_label('output',1,'PosGPS');
      | port_label('output',2,'gravity');
      | port_label('output',3,'TempC');
      | port_label('output',4,'AirPressure');
      | port_label('output',5,'Rho');
      | port_label('output',6,'Windb');
      | port_label('output',7,'Wind');
  __InputSSForSFun__ : Subsystem
  __OutputSSForSFun__ : Subsystem
  Environment Model Bus : Outport
  wires:
  6DOF Bus/1 -> __InputSSForSFun__/1(6DOF Bus)
  __InputSSForSFun__/1(__UniqueOutportName__1__) -> Environment Model_sfcn/1
  __InputSSForSFun__/2(__UniqueOutportName__2__) -> Environment Model_sfcn/2
  __InputSSForSFun__/3(__UniqueOutportName__3__) -> Environment Model_sfcn/3
  __InputSSForSFun__/4(__UniqueOutportName__4__) -> Environment Model_sfcn/4
  __InputSSForSFun__/5(__UniqueOutportName__5__) -> Environment Model_sfcn/5
  __InputSSForSFun__/6(__UniqueOutportName__6__) -> Environment Model_sfcn/6
  __InputSSForSFun__/7(__UniqueOutportName__7__) -> Environment Model_sfcn/7
  Environment Model_sfcn/1 -> __OutputSSForSFun__/1(__UniqueInportName__1__)
  Environment Model_sfcn/2 -> __OutputSSForSFun__/2(__UniqueInportName__2__)
  Environment Model_sfcn/3 -> __OutputSSForSFun__/3(__UniqueInportName__3__)
  Environment Model_sfcn/4 -> __OutputSSForSFun__/4(__UniqueInportName__4__)
  Environment Model_sfcn/5 -> __OutputSSForSFun__/5(__UniqueInportName__5__)
  Environment Model_sfcn/6 -> __OutputSSForSFun__/6(__UniqueInportName__6__)
  Environment Model_sfcn/7 -> __OutputSSForSFun__/7(__UniqueInportName__7__)
  __OutputSSForSFun__/1(Environment Model Bus) -> Environment Model Bus/1

== system CopterSim3DEnvironment/Quadcopter Dynamics/Fail Model ==
  6DOF Bus : Inport
  Fail Model_sfcn : S-Function  FunctionName=Fail_sf  Parameters=sfcnParam1, sfcnParam2, sfcnParam3  SFunctionModules=""  SFunctionDeploymentMode=off  EnableBusSupport=off  mask{rtw_sf_name=Fail_sf, showVar=off, sfcnParam1=sfcnParam1, sfcnParam2=sfcnParam2, sfcnParam3=sfcnParam3}
      mask prompts: rtw_sf_name "Simulink:masks:GenSFuncName_MP"; showVar "Simulink:masks:GenSFuncShowModuleList_MP"; sfcnParam1 "ModelParam_uavJ:"; sfcnParam2 "ModelParam_uavMass:"; sfcnParam3 "ModelParam_uavR:"
      mask help: Simulink:masks:GenSFuncDesc_MD
      mask init: same as CopterSim3DEnvironment/Quadcopter Dynamics/Battery Model/Battery Model_sfcn
      settings: CopyFcn=|
      | if ~strcmp(get_param(gcb,'Linkstatus'),'none') && ...
      | ~strcmp(get_param(gcb,'Linkstatus'),'implicit')
      |   set_param(gcb,'LinkStatus','none');
      | end
      mask Help: eval('feval(''rtwprivate'',''rtwhelpview'',''rtw_sfcn_block'')');
      mask Display:
      | port_label('input',1,'Ve');
      | port_label('input',2,'Xe');
      | port_label('input',3,'Eular(rad)');
      | port_label('input',4,'DCM');
      | port_label('input',5,'Vb');
      | port_label('input',6,'wb');
      | port_label('input',7,'dwb/dt');
      | port_label('output',1,'m');
      | port_label('output',2,'J');
      | port_label('output',3,'dM');
  __InputSSForSFun__ : Subsystem
  __OutputSSForSFun__ : Subsystem
  Fail Model Bus : Outport
  wires:
  6DOF Bus/1 -> __InputSSForSFun__/1(6DOF Bus)
  __InputSSForSFun__/1(__UniqueOutportName__1__) -> Fail Model_sfcn/1
  __InputSSForSFun__/2(__UniqueOutportName__2__) -> Fail Model_sfcn/2
  __InputSSForSFun__/3(__UniqueOutportName__3__) -> Fail Model_sfcn/3
  __InputSSForSFun__/4(__UniqueOutportName__4__) -> Fail Model_sfcn/4
  __InputSSForSFun__/5(__UniqueOutportName__5__) -> Fail Model_sfcn/5
  __InputSSForSFun__/6(__UniqueOutportName__6__) -> Fail Model_sfcn/6
  __InputSSForSFun__/7(__UniqueOutportName__7__) -> Fail Model_sfcn/7
  Fail Model_sfcn/1 -> __OutputSSForSFun__/1(__UniqueInportName__1__)
  Fail Model_sfcn/2 -> __OutputSSForSFun__/2(__UniqueInportName__2__)
  Fail Model_sfcn/3 -> __OutputSSForSFun__/3(__UniqueInportName__3__)
  __OutputSSForSFun__/1(Fail Model Bus) -> Fail Model Bus/1

== system CopterSim3DEnvironment/Quadcopter Dynamics/Force and Moment Model ==
  MotorRads : Inport
  Environment Model Bus : Inport  Port=2
  6DOF Bus : Inport  Port=3
  Fail Model Bus : Inport  Port=4
  "tZ " : Inport  Port=5
  Force and Moment Model_sfcn : S-Function  FunctionName=Force_sf  Parameters=sfcnParam1, sfcnParam2, sfcnParam3, sfcnParam4, sfcnParam5, sfcnParam6, sfcnParam7, sfcnParam8  SFunctionModules=""  SFunctionDeploymentMode=off  EnableBusSupport=off  mask{rtw_sf_name=Force_sf, showVar=off, sfcnParam1=sfcnParam1, sfcnParam2=sfcnParam2, sfcnParam3=sfcnParam3, sfcnParam4=sfcnParam4, sfcnParam5=sfcnParam5, sfcnParam6=sfcnParam6, sfcnParam7=sfcnParam7, sfcnParam8=sfcnParam8}
      mask prompts: rtw_sf_name "Simulink:masks:GenSFuncName_MP"; showVar "Simulink:masks:GenSFuncShowModuleList_MP"; sfcnParam1 "ModelParam_motorJm:"; sfcnParam2 "ModelParam_rotorCm:"; sfcnParam3 "ModelParam_rotorCt:"; sfcnParam4 "ModelParam_uavCCm:"; sfcnParam5 "ModelParam_uavCd:"; sfcnParam6 "ModelParam_uavDearo:"; sfcnParam7 "ModelParam_uavR:"; sfcnParam8 "ModelParam_uavType:"
      mask help: Simulink:masks:GenSFuncDesc_MD
      mask init: same as CopterSim3DEnvironment/Quadcopter Dynamics/Battery Model/Battery Model_sfcn
      settings: CopyFcn=|
      | if ~strcmp(get_param(gcb,'Linkstatus'),'none') && ...
      | ~strcmp(get_param(gcb,'Linkstatus'),'implicit')
      |   set_param(gcb,'LinkStatus','none');
      | end
      mask Help: eval('feval(''rtwprivate'',''rtwhelpview'',''rtw_sfcn_block'')');
      mask Display:
      | port_label('input',1,'MotorRads');
      | port_label('input',2,'PosGPS');
      | port_label('input',3,'gravity');
      | port_label('input',4,'TempC');
      | port_label('input',5,'AirPressure');
      | port_label('input',6,'Rho');
      | port_label('input',7,'Windb');
      | port_label('input',8,'Wind');
      | port_label('input',9,'Ve');
      | port_label('input',10,'Xe');
      | port_label('input',11,'Eular(rad)');
      | port_label('input',12,'DCM');
      | port_label('input',13,'Vb');
      | port_label('input',14,'wb');
      | port_label('input',15,'dwb/dt');
      | port_label('input',16,'m');
      | port_label('input',17,'J');
      | port_label('input',18,'dM');
      | port_label('input',19,'tZ ');
      | port_label('output',1,'Fb');
      | port_label('output',2,'Mb');
      | port_label('output',3,'landed');
  __InputSSForSFun__ : Subsystem
  __OutputSSForSFun__ : Subsystem
  Force and Moment Model Bus : Outport
  wires:
  MotorRads/1 -> __InputSSForSFun__/1(MotorRads)
  Environment Model Bus/1 -> __InputSSForSFun__/2(Environment Model Bus)
  6DOF Bus/1 -> __InputSSForSFun__/3(6DOF Bus)
  Fail Model Bus/1 -> __InputSSForSFun__/4(Fail Model Bus)
  "tZ "/1 -> __InputSSForSFun__/5("tZ ")
  __InputSSForSFun__/1(__UniqueOutportName__1__) -> Force and Moment Model_sfcn/1
  __InputSSForSFun__/2(__UniqueOutportName__2__) -> Force and Moment Model_sfcn/2
  __InputSSForSFun__/3(__UniqueOutportName__3__) -> Force and Moment Model_sfcn/3
  __InputSSForSFun__/4(__UniqueOutportName__4__) -> Force and Moment Model_sfcn/4
  __InputSSForSFun__/5(__UniqueOutportName__5__) -> Force and Moment Model_sfcn/5
  __InputSSForSFun__/6(__UniqueOutportName__6__) -> Force and Moment Model_sfcn/6
  __InputSSForSFun__/7(__UniqueOutportName__7__) -> Force and Moment Model_sfcn/7
  __InputSSForSFun__/8(__UniqueOutportName__8__) -> Force and Moment Model_sfcn/8
  __InputSSForSFun__/9(__UniqueOutportName__9__) -> Force and Moment Model_sfcn/9
  __InputSSForSFun__/10(__UniqueOutportName__10__) -> Force and Moment Model_sfcn/10
  __InputSSForSFun__/11(__UniqueOutportName__11__) -> Force and Moment Model_sfcn/11
  __InputSSForSFun__/12(__UniqueOutportName__12__) -> Force and Moment Model_sfcn/12
  __InputSSForSFun__/13(__UniqueOutportName__13__) -> Force and Moment Model_sfcn/13
  __InputSSForSFun__/14(__UniqueOutportName__14__) -> Force and Moment Model_sfcn/14
  __InputSSForSFun__/15(__UniqueOutportName__15__) -> Force and Moment Model_sfcn/15
  __InputSSForSFun__/16(__UniqueOutportName__16__) -> Force and Moment Model_sfcn/16
  __InputSSForSFun__/17(__UniqueOutportName__17__) -> Force and Moment Model_sfcn/17
  __InputSSForSFun__/18(__UniqueOutportName__18__) -> Force and Moment Model_sfcn/18
  __InputSSForSFun__/19(__UniqueOutportName__19__) -> Force and Moment Model_sfcn/19
  Force and Moment Model_sfcn/1 -> __OutputSSForSFun__/1(__UniqueInportName__1__)
  Force and Moment Model_sfcn/2 -> __OutputSSForSFun__/2(__UniqueInportName__2__)
  Force and Moment Model_sfcn/3 -> __OutputSSForSFun__/3(__UniqueInportName__3__)
  __OutputSSForSFun__/1(Force and Moment Model Bus) -> Force and Moment Model Bus/1

== system CopterSim3DEnvironment/Quadcopter Dynamics/Motor Model ==
  Battery Model Bus : Inport
  Motor Model_sfcn : S-Function  FunctionName=Motor_sf  Parameters=sfcnParam1, sfcnParam2, sfcnParam3, sfcnParam4, sfcnParam5  SFunctionModules=""  SFunctionDeploymentMode=off  EnableBusSupport=off  mask{rtw_sf_name=Motor_sf, showVar=off, sfcnParam1=sfcnParam1, sfcnParam2=sfcnParam2, sfcnParam3=sfcnParam3, sfcnParam4=sfcnParam4, sfcnParam5=sfcnParam5}
      mask prompts: rtw_sf_name "Simulink:masks:GenSFuncName_MP"; showVar "Simulink:masks:GenSFuncShowModuleList_MP"; sfcnParam1 "ModelInit_RPM:"; sfcnParam2 "ModelParam_motorCr:"; sfcnParam3 "ModelParam_motorMinThr:"; sfcnParam4 "ModelParam_motorT:"; sfcnParam5 "ModelParam_motorWb:"
      mask help: Simulink:masks:GenSFuncDesc_MD
      mask init: same as CopterSim3DEnvironment/Quadcopter Dynamics/Battery Model/Battery Model_sfcn
      settings: CopyFcn=|
      | if ~strcmp(get_param(gcb,'Linkstatus'),'none') && ...
      | ~strcmp(get_param(gcb,'Linkstatus'),'implicit')
      |   set_param(gcb,'LinkStatus','none');
      | end
      mask Help: eval('feval(''rtwprivate'',''rtwhelpview'',''rtw_sfcn_block'')');
      mask Display:
      | port_label('input',1,'PWMOut');
      | port_label('input',2,'cellVol');
      | port_label('input',3,'remCapa');
      | port_label('output',1,'MotorRads');
  __InputSSForSFun__ : Subsystem
  __OutputSSForSFun__ : Subsystem
  MotorRads : Outport
  wires:
  Battery Model Bus/1 -> __InputSSForSFun__/1(Battery Model Bus)
  __InputSSForSFun__/1(__UniqueOutportName__1__) -> Motor Model_sfcn/1
  __InputSSForSFun__/2(__UniqueOutportName__2__) -> Motor Model_sfcn/2
  __InputSSForSFun__/3(__UniqueOutportName__3__) -> Motor Model_sfcn/3
  Motor Model_sfcn/1 -> __OutputSSForSFun__/1(__UniqueInportName__1__)
  __OutputSSForSFun__/1(MotorRads) -> MotorRads/1
